simulink model "CounterDroneSystem"  (R2026a)
settings: Solver=FixedStepAuto  StopTime=20  FixedStep=0.001
libraries: simulink x9
settings Model: Creator=ACER  LastModifiedBy=ACER

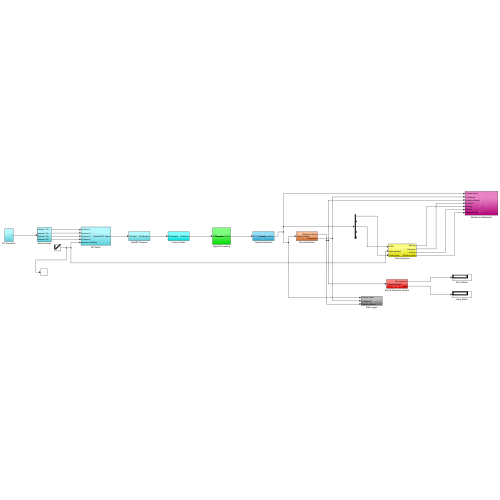
[thumbnail: Simulink's stored preview of the top-level diagram]
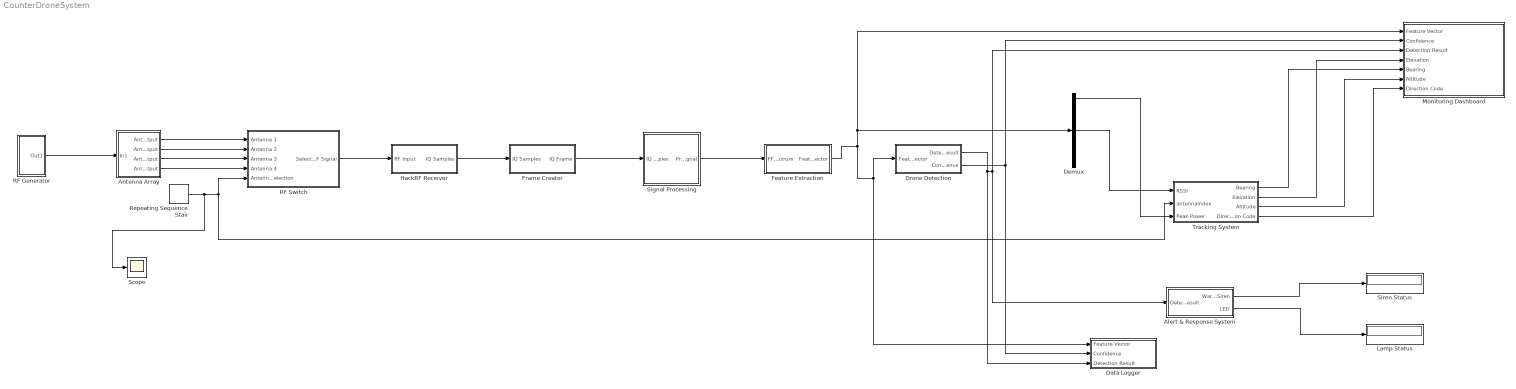
== system CounterDroneSystem ==
  Alert & Response System : Subsystem
  Antenna Array : Subsystem
  Data Logger : Subsystem
  Demux : Demux  Outputs=5
  Drone Detection : Subsystem
  Feature Extraction : Subsystem
  Frame Creator : Subsystem
  HackRF Receiver : Subsystem
  Lamp Status : Display
  Monitoring Dashboard : Subsystem
  RF Generator : Subsystem
  RF Switch : Subsystem
  Repeating Sequence Stair : simulink/Sources/Repeating Sequence Stair  OutValues=[1 2 3 4]  tsamp=5  OutMin=[]  OutMax=[]  OutDataTypeStr=double  OutputDataTypeScalingMode=double  OutDataType=fixdt(0,8)  ConRadixGroup=Best Precision: Vector-wise  OutScaling=2^-12
  Scope : Scope
      settings: ActiveDisplayYMinimum=0.75000000000000011  ActiveDisplayYMaximum=3.25
  Signal Processing : Subsystem
  Siren Status : Display
  Tracking System : Subsystem
  wires:
  RF Generator/1(Out1) -> Antenna Array/1(In1)
  Antenna Array/1(Antenna 1 Output) -> RF Switch/1(Antenna 1)
  Antenna Array/2(Antenna 2 Output) -> RF Switch/2(Antenna 2)
  Signal Processing/1(Processed Signal) -> Feature Extraction/1(FFT Spectrum)
  Feature Extraction/1(Feature Vector) -> Monitoring Dashboard/1(Feature Vector), Demux/1, Data Logger/1(Feature Vector), Drone Detection/1(Feature Vector)
  Drone Detection/2(Confidence) -> Data Logger/2(Confidence), Monitoring Dashboard/2(Confidence)
  Drone Detection/1(Detection Result) -> Data Logger/3(Detection Result), Monitoring Dashboard/3(Detection Result), Alert & Response System/1(Detection Result)
  Tracking System/2(Elevation) -> Monitoring Dashboard/4(Elevation)
  Tracking System/3(" Altitude") -> Monitoring Dashboard/6(Altitude)
  Alert & Response System/1(Warning Siren) -> Siren Status/1
  Alert & Response System/2(" LED") -> Lamp Status/1
  Demux/1 -> Tracking System/3(Peak Power)
  Demux/3 -> Tracking System/1(RSSI)
  Repeating Sequence Stair/1 -> Scope/1, Tracking System/2(antennaIndex), RF Switch/5(Antenna Selection)
  Antenna Array/3(Antenna 3 Output) -> RF Switch/3(Antenna 3)
  Antenna Array/4(Antenna 4 Output) -> RF Switch/4(Antenna 4)
  Frame Creator/1(IQ Frame) -> Signal Processing/1(IQ Samples)
  Tracking System/1(Bearing) -> Monitoring Dashboard/5(Bearing)
  Tracking System/4(Direction Code) -> Monitoring Dashboard/7(Direction Code)
  RF Switch/1(Selected RF Signal) -> HackRF Receiver/1(RF Input)
  HackRF Receiver/1(IQ Samples) -> Frame Creator/1(IQ Samples)

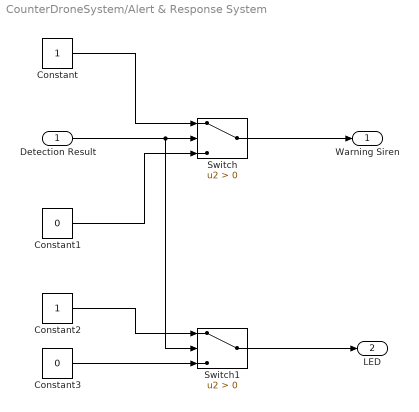
== system CounterDroneSystem/Alert & Response System ==
  Detection Result : Inport
  Constant : Constant
  Constant1 : Constant  Value=0
  Constant2 : Constant
  Constant3 : Constant  Value=0
  Switch : Switch  Criteria=u2 > Threshold  SaturateOnIntegerOverflow=off  InputSameDT=off
  Switch1 : Switch  Criteria=u2 > Threshold  SaturateOnIntegerOverflow=off  InputSameDT=off
  Warning Siren : Outport
  " LED" : Outport  Port=2
  wires:
  Detection Result/1 -> Switch1/2, Switch/2
  Constant/1 -> Switch/1
  Constant1/1 -> Switch/3
  Switch/1 -> Warning Siren/1
  Constant2/1 -> Switch1/1
  Constant3/1 -> Switch1/3
  Switch1/1 -> " LED"/1

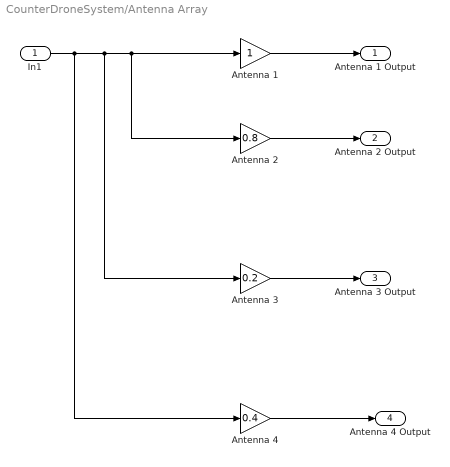
== system CounterDroneSystem/Antenna Array ==
  In1 : Inport
  Antenna 1 : Gain
  Antenna 2 : Gain  Gain=0.8
  Antenna 3 : Gain  Gain=0.2
  Antenna 4 : Gain  Gain=0.4
  Antenna 1 Output : Outport
  Antenna 2 Output : Outport  Port=2
  Antenna 3 Output : Outport  Port=3
  Antenna 4 Output : Outport  Port=4
  wires:
  Antenna 2/1 -> Antenna 2 Output/1
  In1/1 -> Antenna 4/1, Antenna 3/1, Antenna 2/1, Antenna 1/1
  Antenna 1/1 -> Antenna 1 Output/1
  Antenna 3/1 -> Antenna 3 Output/1
  Antenna 4/1 -> Antenna 4 Output/1

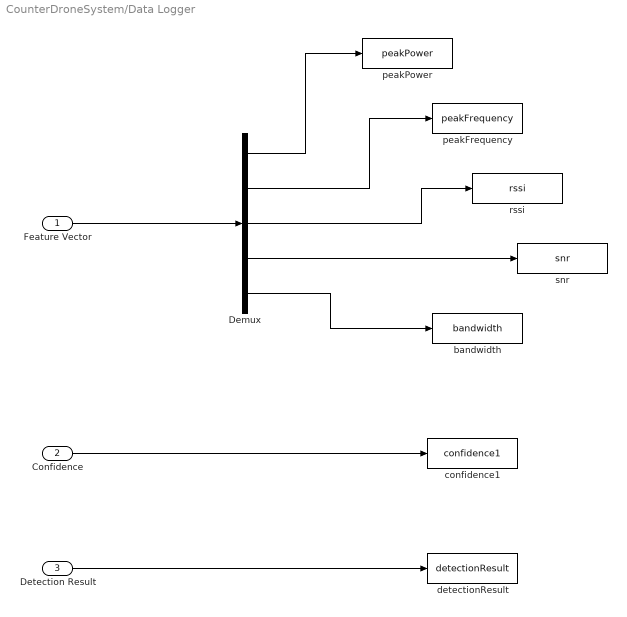
== system CounterDroneSystem/Data Logger ==
  Feature Vector : Inport
  Confidence : Inport  Port=2
  Detection Result : Inport  Port=3
  Demux : Demux  Outputs=5
  bandwidth : ToWorkspace  VariableName=bandwidth  SampleTime=-1
  confidence1 : ToWorkspace  VariableName=confidence1  SampleTime=-1
  detectionResult : ToWorkspace  VariableName=detectionResult  SampleTime=-1
  peakFrequency : ToWorkspace  VariableName=peakFrequency  SampleTime=-1
  peakPower : ToWorkspace  VariableName=peakPower  SampleTime=-1
  rssi : ToWorkspace  VariableName=rssi  SampleTime=-1
  snr : ToWorkspace  VariableName=snr  SampleTime=-1
  wires:
  Feature Vector/1 -> Demux/1
  Demux/1 -> peakPower/1
  Demux/2 -> peakFrequency/1
  Demux/3 -> rssi/1
  Demux/4 -> snr/1
  Demux/5 -> bandwidth/1
  Confidence/1 -> confidence1/1
  Detection Result/1 -> detectionResult/1

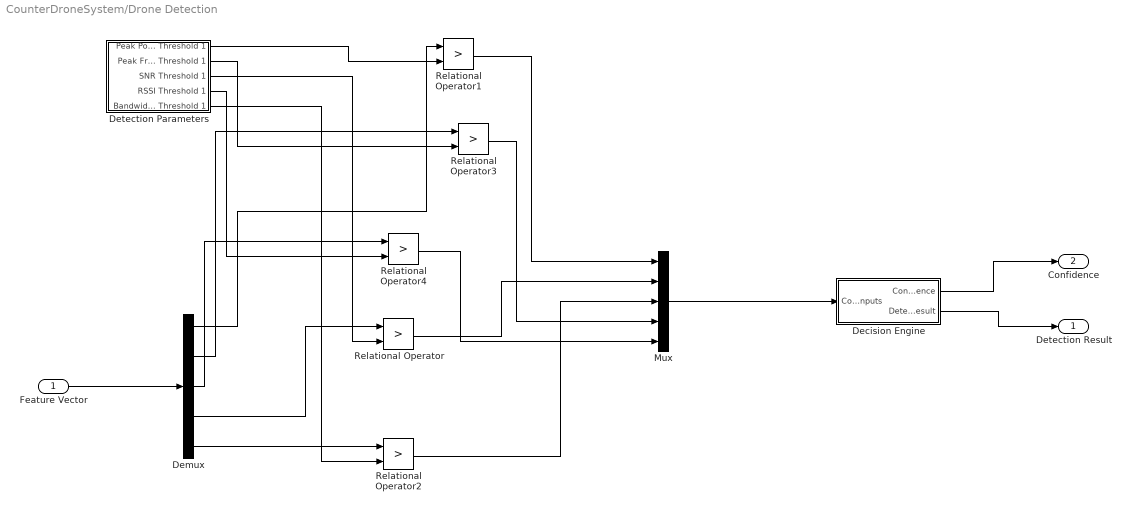
== system CounterDroneSystem/Drone Detection ==
  Feature Vector : Inport
  Decision Engine : Subsystem
  Demux : Demux  Outputs=5
  Detection Parameters : Subsystem
  Mux : Mux  Inputs=5
  Relational Operator{,1..4} (5 alike) : RelationalOperator  Operator=>  OutDataTypeStr=boolean  RndMeth=Simplest  InputSameDT=off
  Detection Result : Outport
  Confidence : Outport  Port=2
  wires:
  Feature Vector/1 -> Demux/1
  Demux/1 -> Relational Operator1/1
  Demux/4 -> Relational Operator/1
  Demux/5 -> Relational Operator2/1
  Relational Operator1/1 -> Mux/1
  Relational Operator/1 -> Mux/2
  Relational Operator2/1 -> Mux/3
  Mux/1 -> Decision Engine/1(Comparator Inputs)
  Decision Engine/1(Confidence) -> Confidence/1
  Decision Engine/2(Detection Result) -> Detection Result/1
  Detection Parameters/1(Peak Power Threshold 1) -> Relational Operator1/2
  Detection Parameters/5(" Bandwidth Threshold 1") -> Relational Operator2/2
  Detection Parameters/3(SNR Threshold 1) -> Relational Operator/2
  Demux/2 -> Relational Operator3/1
  Detection Parameters/2(Peak Frequency Threshold 1) -> Relational Operator3/2
  Relational Operator3/1 -> Mux/4
  Relational Operator4/1 -> Mux/5
  Detection Parameters/4(RSSI Threshold 1) -> Relational Operator4/2
  Demux/3 -> Relational Operator4/1

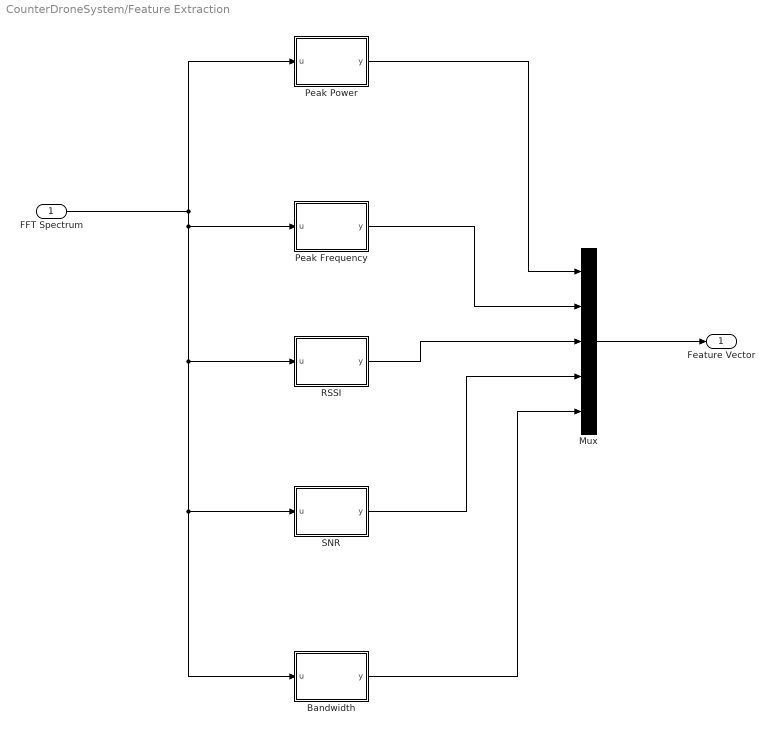
== system CounterDroneSystem/Feature Extraction ==
  FFT Spectrum : Inport
  Bandwidth : MATLAB Function  TreatAsAtomicUnit=on
  Mux : Mux  Inputs=5
  Peak Frequency : MATLAB Function  TreatAsAtomicUnit=on
  Peak Power : MATLAB Function  TreatAsAtomicUnit=on
  RSSI : MATLAB Function  TreatAsAtomicUnit=on
  SNR : MATLAB Function  TreatAsAtomicUnit=on
  Feature Vector : Outport
  wires:
  FFT Spectrum/1 -> Peak Frequency/1(u), Bandwidth/1(u), SNR/1(u), RSSI/1(u), Peak Power/1(u)
  Mux/1 -> Feature Vector/1
  RSSI/1(y) -> Mux/3
  SNR/1(y) -> Mux/4
  Bandwidth/1(y) -> Mux/5
  Peak Frequency/1(y) -> Mux/2
  Peak Power/1(y) -> Mux/1

== system CounterDroneSystem/Frame Creator ==
  IQ Samples : Inport
  Buffer : Buffer  N=256  OutputFrames=off
  IQ Frame : Outport
  wires:
  IQ Samples/1 -> Buffer/1
  Buffer/1 -> IQ Frame/1

== system CounterDroneSystem/HackRF Receiver ==
  RF Input : Inport
  LNA : Gain  Gain=10
  IQ Samples : Outport
  wires:
  RF Input/1 -> LNA/1
  LNA/1 -> IQ Samples/1

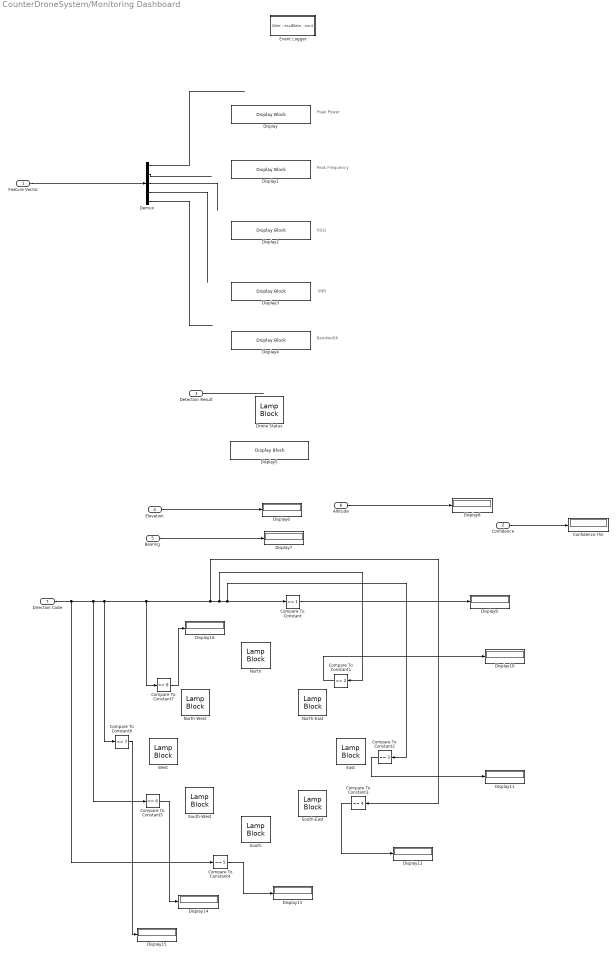
== system CounterDroneSystem/Monitoring Dashboard ==
  note: Peak Frequency
  note: Bandwidth
  note: SNR
  note: Peak Power
  note: RSSI
  Feature Vector : Inport
  Confidence : Inport  Port=2
  Detection Result : Inport  Port=3
  Elevation : Inport  Port=4
  Bearing : Inport  Port=5
  Altitude : Inport  Port=6
  Direction Code : Inport  Port=7
  " Confidence (%)" : Display
  Compare To Constant : simulink/Logic and Bit Operations/Compare To Constant  relop===  const=1  OutDataTypeStr=boolean
  Compare To Constant1 : simulink/Logic and Bit Operations/Compare To Constant  relop===  const=2  OutDataTypeStr=boolean
  Compare To Constant2 : simulink/Logic and Bit Operations/Compare To Constant  relop===  const=3  OutDataTypeStr=boolean
  Compare To Constant3 : simulink/Logic and Bit Operations/Compare To Constant  relop===  const=4  OutDataTypeStr=boolean
  Compare To Constant4 : simulink/Logic and Bit Operations/Compare To Constant  relop===  const=5  OutDataTypeStr=boolean
  Compare To Constant5 : simulink/Logic and Bit Operations/Compare To Constant  relop===  const=6  OutDataTypeStr=boolean
  Compare To Constant6 : simulink/Logic and Bit Operations/Compare To Constant  relop===  const=7  OutDataTypeStr=boolean
  Compare To Constant7 : simulink/Logic and Bit Operations/Compare To Constant  relop===  const=8  OutDataTypeStr=boolean
  Demux : Demux  Outputs=5
  Display{,1..5} (6 alike) : DisplayBlock  LabelPosition=Hide  Transparency=1  GridColor=[0.502, 0.502, 0.502]
  Display{6..16} (11 alike) : Display
  Drone Status : LampBlock  LabelPosition=Hide  DefaultColor=[192.0, 192.0, 192.0]
  East : LampBlock  LabelPosition=Hide  DefaultColor=[192.0, 192.0, 192.0]
  Event Logger : Subsystem
  North : LampBlock  LabelPosition=Hide  DefaultColor=[192.0, 192.0, 192.0]
  North-East : LampBlock  LabelPosition=Hide  DefaultColor=[192.0, 192.0, 192.0]
  North-West : LampBlock  LabelPosition=Hide  DefaultColor=[192.0, 192.0, 192.0]
  South : LampBlock  LabelPosition=Hide  DefaultColor=[192.0, 192.0, 192.0]
  South-East : LampBlock  LabelPosition=Hide  DefaultColor=[192.0, 192.0, 192.0]
  South-West : LampBlock  LabelPosition=Hide  DefaultColor=[192.0, 192.0, 192.0]
  West : LampBlock  LabelPosition=Hide  DefaultColor=[192.0, 192.0, 192.0]
  wires:
  Demux/2 -> ?
  Demux/1 -> ?
  Demux/5 -> ?
  Demux/3 -> ?
  Demux/4 -> ?
  Feature Vector/1 -> Demux/1
  Confidence/1 -> " Confidence (%)"/1
  Detection Result/1 -> ?
  Elevation/1 -> Display6/1
  Bearing/1 -> Display7/1
  Altitude/1 -> Display8/1
  Direction Code/1 -> Compare To Constant4/1, Compare To Constant5/1, Compare To Constant3/1, Compare To Constant1/1, Compare To Constant2/1, Compare To Constant/1, Compare To Constant7/1, Compare To Constant6/1
  Compare To Constant/1 -> Display9/1
  Compare To Constant1/1 -> Display10/1
  Compare To Constant2/1 -> Display11/1
  Compare To Constant3/1 -> Display12/1
  Compare To Constant4/1 -> Display13/1
  Compare To Constant5/1 -> Display14/1
  Compare To Constant6/1 -> Display15/1
  Compare To Constant7/1 -> Display16/1

== system CounterDroneSystem/RF Generator ==
  Random Number : RandomNumber  Variance=0.01  SampleTime=0.001
  Sine Wave : Sin  Amplitude=10  Frequency=1000  SampleTime=0.001
  Sum : Sum  Inputs=|++
  Out1 : Outport
  wires:
  Sine Wave/1 -> Sum/1
  Sum/1 -> Out1/1
  Random Number/1 -> Sum/2

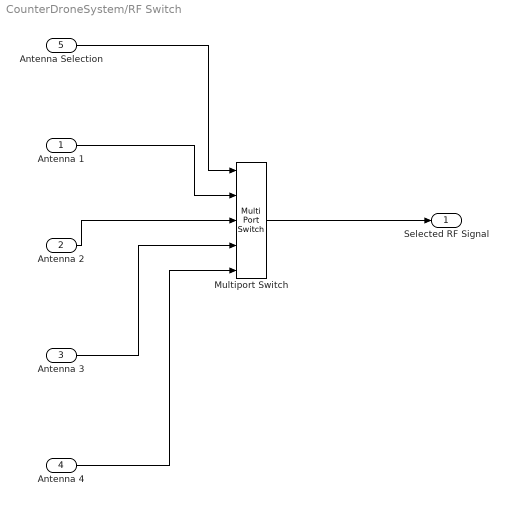
== system CounterDroneSystem/RF Switch ==
  Antenna 1 : Inport
  Antenna 2 : Inport  Port=2
  Antenna 3 : Inport  Port=3
  Antenna 4 : Inport  Port=4
  Antenna Selection : Inport  Port=5
  Multiport Switch : MultiPortSwitch  Inputs=4  SaturateOnIntegerOverflow=off  InputSameDT=off
  Selected RF Signal : Outport
  wires:
  Antenna Selection/1 -> Multiport Switch/1
  Antenna 1/1 -> Multiport Switch/2
  Antenna 2/1 -> Multiport Switch/3
  Antenna 3/1 -> Multiport Switch/4
  Antenna 4/1 -> Multiport Switch/5
  Multiport Switch/1 -> Selected RF Signal/1

== system CounterDroneSystem/Signal Processing ==
  IQ Samples : Inport
  Array Plot : ArrayPlot  WindowPosition=[19.000000,179.000000,800.000000,500.000000,]  ScopeFrameLocation=window  AxesScaling=Manual  Title=RF Power Spectrum  YLimits=[-529.6101893004114 1954.8544106995882]
  Band Pass Filter : Subsystem
  Power Estimation : MATLAB Function  TreatAsAtomicUnit=on
  Processed Signal : Outport
  wires:
  IQ Samples/1 -> Band Pass Filter/1(IQ Samples)
  Band Pass Filter/1(FFT Spectrum) -> Power Estimation/1(u)
  Power Estimation/1(y) -> Array Plot/1, Processed Signal/1

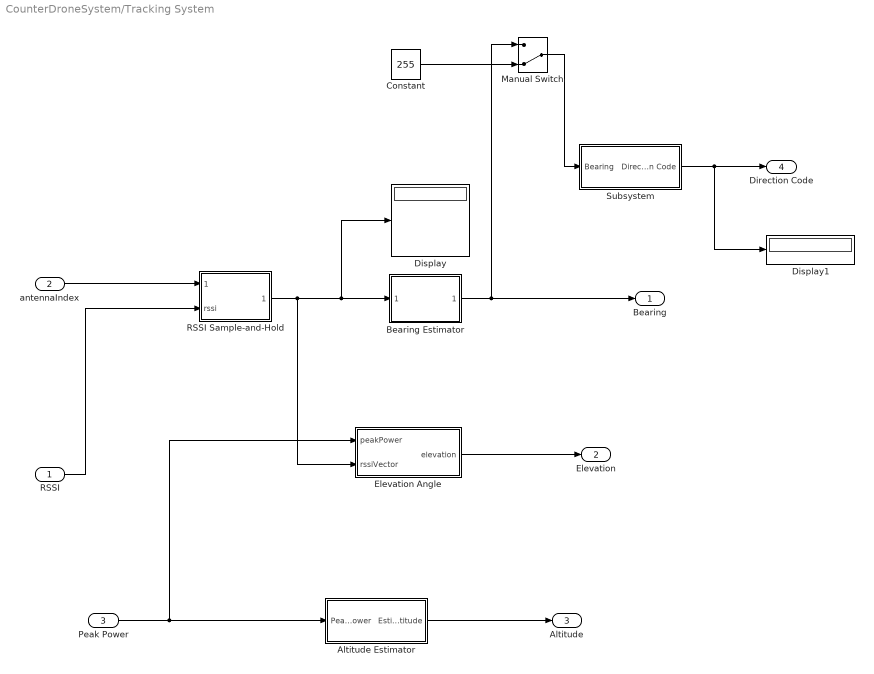
== system CounterDroneSystem/Tracking System ==
  RSSI : Inport
  antennaIndex : Inport  Port=2
  Peak Power : Inport  Port=3
  Altitude Estimator : Subsystem
  Bearing Estimator : MATLAB Function  TreatAsAtomicUnit=on
  Constant : Constant  Value=255
  Display : Display
  Display1 : Display
  Elevation Angle : MATLAB Function  TreatAsAtomicUnit=on
  Manual Switch : ManualSwitch  CurrentSetting=0
  RSSI Sample-and-Hold : MATLAB Function  TreatAsAtomicUnit=on
  Subsystem : Subsystem
  Bearing : Outport
  Elevation : Outport  Port=2
  " Altitude" : Outport  Port=3
  Direction Code : Outport  Port=4
  wires:
  Altitude Estimator/1(Estimated Altitude) -> " Altitude"/1
  Peak Power/1 -> Elevation Angle/1(peakPower), Altitude Estimator/1(Peak power)
  antennaIndex/1 -> RSSI Sample-and-Hold/1(antennaIndex)
  RSSI/1 -> RSSI Sample-and-Hold/2(rssi)
  RSSI Sample-and-Hold/1(rssiVector) -> Elevation Angle/2(rssiVector), Display/1, Bearing Estimator/1(rssiVector)
  Bearing Estimator/1(bearing) -> Bearing/1, Manual Switch/1
  Elevation Angle/1(elevation) -> Elevation/1
  Subsystem/1(Direction Code) -> Display1/1, Direction Code/1
  Constant/1 -> Manual Switch/2
  Manual Switch/1 -> Subsystem/1(Bearing)

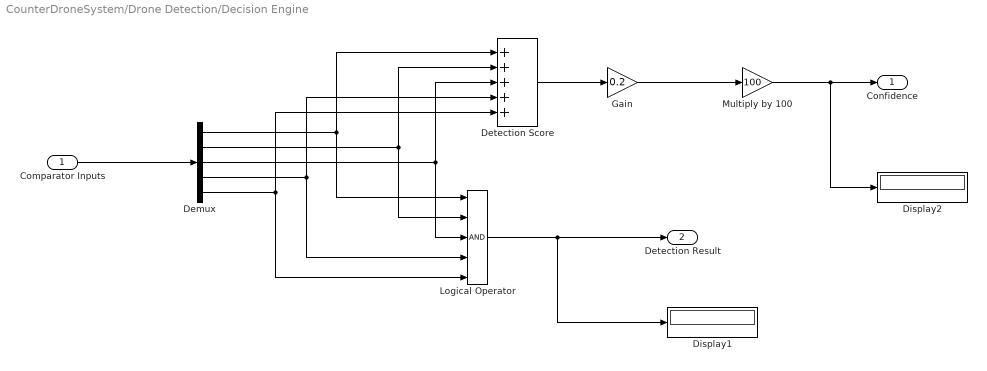
== system CounterDroneSystem/Drone Detection/Decision Engine ==
  Comparator Inputs : Inport
  Demux : Demux  Outputs=5
  Detection Score : Sum  Inputs=+++++
  Display1 : Display
  Display2 : Display
  Gain : Gain  Gain=0.2
  Logical Operator : Logic  Inputs=5  AllPortsSameDT=off  OutDataTypeStr=boolean
  Multiply by 100 : Gain  Gain=100
  Confidence : Outport
  Detection Result : Outport  Port=2
  wires:
  Multiply by 100/1 -> Display2/1, Confidence/1
  Demux/3 -> Logical Operator/3, Detection Score/3
  Logical Operator/1 -> Display1/1, Detection Result/1
  Gain/1 -> Multiply by 100/1
  Demux/2 -> Logical Operator/2, Detection Score/2
  Detection Score/1 -> Gain/1
  Demux/1 -> Logical Operator/1, Detection Score/1
  Comparator Inputs/1 -> Demux/1
  Demux/4 -> Logical Operator/4, Detection Score/4
  Demux/5 -> Logical Operator/5, Detection Score/5

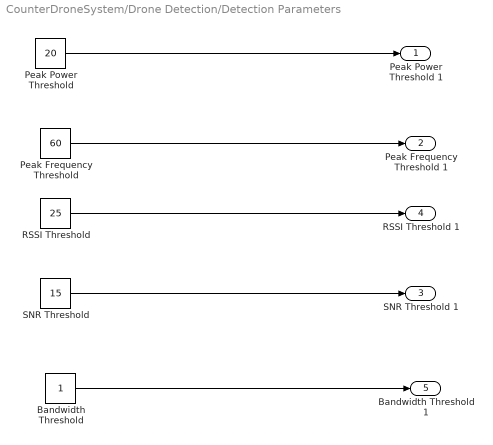
== system CounterDroneSystem/Drone Detection/Detection Parameters ==
  Bandwidth Threshold : Constant
  Peak Frequency Threshold : Constant  Value=60
  Peak Power Threshold : Constant  Value=20
  RSSI Threshold : Constant  Value=25
  SNR Threshold : Constant  Value=15
  Peak Power Threshold 1 : Outport
  Peak Frequency Threshold 1 : Outport  Port=2
  SNR Threshold 1 : Outport  Port=3
  RSSI Threshold 1 : Outport  Port=4
  " Bandwidth Threshold 1" : Outport  Port=5
  wires:
  Peak Power Threshold/1 -> Peak Power Threshold 1/1
  RSSI Threshold/1 -> RSSI Threshold 1/1
  SNR Threshold/1 -> SNR Threshold 1/1
  Bandwidth Threshold/1 -> " Bandwidth Threshold 1"/1
  Peak Frequency Threshold/1 -> Peak Frequency Threshold 1/1

== system CounterDroneSystem/Monitoring Dashboard/Event Logger ==
  Detection Result : Inport
  Detection Count : Outport
  wires:
  Detection Result/1 -> Detection Count/1

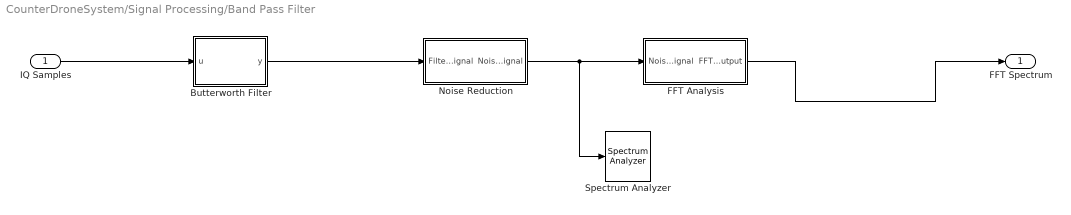
== system CounterDroneSystem/Signal Processing/Band Pass Filter ==
  IQ Samples : Inport
  Butterworth Filter : MATLAB Function  TreatAsAtomicUnit=on
  FFT Analysis : Subsystem
  Noise Reduction : Subsystem
  Spectrum Analyzer : SpectrumAnalyzer  WindowPosition=[1.000000,1.000000,1536.000000,841.000000,]  Visible=on  ScopeFrameLocation=window  WindowInvariantSamplesPerUpdate=on  Span=1000  StartFrequency=-500  StopFrequency=500  YLimits=[-35.2084 48.8632]
  FFT Spectrum : Outport
  wires:
  IQ Samples/1 -> Butterworth Filter/1(u)
  Butterworth Filter/1(y) -> Noise Reduction/1(Filtered Signal)
  Noise Reduction/1(Noise Reduced Signal) -> Spectrum Analyzer/1, FFT Analysis/1(Noise Reduced Signal)
  FFT Analysis/1(FFT Output) -> FFT Spectrum/1

== system CounterDroneSystem/Tracking System/Altitude Estimator ==
  Peak power : Inport
  Bias : Bias  Bias=0.05  SaturateOnIntegerOverflow=off
  Gain : Gain  Gain=0.5
  Saturation : Saturate  UpperLimit=120  LowerLimit=0
  Estimated Altitude : Outport
  wires:
  Peak power/1 -> Gain/1
  Gain/1 -> Bias/1
  Bias/1 -> Saturation/1
  Saturation/1 -> Estimated Altitude/1

== system CounterDroneSystem/Tracking System/Subsystem ==
  Bearing : Inport
  MATLAB Function : MATLAB Function  TreatAsAtomicUnit=on
  Direction Code : Outport
  wires:
  Bearing/1 -> MATLAB Function/1(bearing)
  MATLAB Function/1(direction) -> Direction Code/1

== system CounterDroneSystem/Signal Processing/Band Pass Filter/FFT Analysis ==
  Noise Reduced Signal : Inport
  FFT Processor : MATLAB Function  TreatAsAtomicUnit=on
  FFT Output : Outport
  wires:
  Noise Reduced Signal/1 -> FFT Processor/1(u)
  FFT Processor/1(y) -> FFT Output/1

== system CounterDroneSystem/Signal Processing/Band Pass Filter/Noise Reduction ==
  Filtered Signal : Inport
  Noise Reduction : MATLAB Function  TreatAsAtomicUnit=on
  Noise Reduced Signal : Outport
  wires:
  Filtered Signal/1 -> Noise Reduction/1(u)
  Noise Reduction/1(y) -> Noise Reduced Signal/1

== matlab function CounterDroneSystem/Signal Processing/Band Pass Filter/Butterworth Filter ==
  data: u input; y output
function y = fcn(u)
%--------------------------------------------------------------------------
% Counter Drone System
% Band Pass Filter
%
% Input  : u  -> IQ Samples
% Output : y  -> Filtered Signal
%
% Current Version:
% Passes the signal directly.
% A real Butterworth Band Pass Filter will be added later.
%--------------------------------------------------------------------------

% Pass the input signal directly
y = u;

end

== matlab function CounterDroneSystem/Signal Processing/Band Pass Filter/FFT Analysis/FFT Processor ==
  data: u input; y output
function y = fcn(u)
%=========================================================
% Counter Drone System
% FFT Processor
%
% Input  : IQ Samples
% Output : Normalized FFT Magnitude Spectrum
%=========================================================

% Convert to column vector
x = u(:);

% Number of samples
N = length(x);

% Compute normalized FFT
X = fft(x)/N;

% Shift zero frequency to center
X = fftshift(X);

% Magnitude spectrum
y = abs(X);

end

== matlab function CounterDroneSystem/Signal Processing/Power Estimation ==
  data: u input; y output
function y = fcn(u)

% Power Spectrum

y = abs(u).^2;

% Remove DC component
y = y - min(y);

end

== matlab function CounterDroneSystem/Tracking System/Subsystem/MATLAB Function ==
  data: bearing input; direction output
function direction = fcn(bearing)

bearing = mod(bearing,360);

if bearing >= 337.5 || bearing < 22.5
    direction = 1;      % North

elseif bearing >=22.5 && bearing <67.5
    direction = 2;      % North-East

elseif bearing >=67.5 && bearing <112.5
    direction = 3;      % East

elseif bearing >=112.5 && bearing <157.5
    direction = 4;      % South-East

elseif bearing >=157.5 && bearing <202.5
    direction = 5;      % South

elseif bearing >=202.5 && bearing <247.5
    direction = 6;      % South-West

elseif bearing >=247.5 && bearing <292.5
    direction = 7;      % West

else
    direction = 8;      % North-West

end

== matlab function CounterDroneSystem/Feature Extraction/Peak Power ==
  data: u input; y output
function y = fcn(u)

% Peak Power in dB

peak = max(u);

y = 10*log10(peak + eps);

end

== matlab function CounterDroneSystem/Feature Extraction/Peak Frequency ==
  data: u input; y output
function y = fcn(u)

[~,idx] = max(abs(u));
y = idx;

end

== matlab function CounterDroneSystem/Feature Extraction/RSSI ==
  data: u input; y output
function y = fcn(u)

y = 10*log10(mean(abs(u).^2)+eps);

end

== matlab function CounterDroneSystem/Feature Extraction/SNR ==
  data: u input; y output
function y = fcn(u)

signal = max(abs(u).^2);
noise = mean(abs(u).^2);

y = 10*log10(signal/(noise+eps));

end

== matlab function CounterDroneSystem/Feature Extraction/Bandwidth ==
  data: u input; y output
function y = fcn(u)

threshold = max(abs(u))*0.5;

index = find(abs(u)>threshold);

y = length(index);

end

== matlab function CounterDroneSystem/Tracking System/RSSI Sample-and-Hold ==
  data: antennaIndex input; rssiVector output; rssi input
function rssiVector = fcn(antennaIndex, rssi)
persistent heldValues lastIndex skipCount
if isempty(heldValues)
    heldValues = zeros(1,4);
    lastIndex = -1;
    skipCount = 0;
end
idx = round(antennaIndex);
if idx ~= lastIndex
    lastIndex = idx;
    skipCount = 2;
end
if idx >= 1 && idx <= 4
    if skipCount > 0
        skipCount = skipCount - 1;
    else
        heldValues(idx) = rssi;
    end
end
rssiVector = heldValues;
end

== matlab function CounterDroneSystem/Signal Processing/Band Pass Filter/Noise Reduction/Noise Reduction ==
  data: u input; y output
function y = fcn(u)
%---------------------------------------------------------
% Counter Drone System
% Noise Reduction
%
% Input  : Filtered Signal
% Output : Noise Reduced Signal
%
% Current Version:
% Passes the signal directly.
% A real denoising algorithm will be added later.
%---------------------------------------------------------

% Pass input directly to output
y = u;

end

== matlab function CounterDroneSystem/Tracking System/Bearing Estimator ==
  data: rssiVector input; bearing output
function bearing = fcn(rssiVector)
angles = [0 90 180 270];
linPower = 10.^(rssiVector/10);
[~, maxIdx] = max(linPower);
leftIdx  = mod(maxIdx-2,4) + 1;
rightIdx = mod(maxIdx,4) + 1;
if linPower(leftIdx) >= linPower(rightIdx)
    neighborIdx = leftIdx;
else
    neighborIdx = rightIdx;
end
w1 = linPower(maxIdx);
w2 = linPower(neighborIdx);
a1 = angles(maxIdx);
a2 = angles(neighborIdx);
diffAngle = a2 - a1;
if diffAngle > 180
    diffAngle = diffAngle - 360;
elseif diffAngle < -180
    diffAngle = diffAngle + 360;
end
fraction = w2 / (w1 + w2 + eps);
bearing = mod(a1 + fraction*diffAngle, 360);
end

== matlab function CounterDroneSystem/Tracking System/Elevation Angle ==
  data: peakPower input; elevation output double; rssiVector input
function elevation = fcn(peakPower, rssiVector)

validRSSI = rssiVector(rssiVector ~= 0);

if numel(validRSSI) < 2
    elevation = 0;
    return;
end

rssiStd = std(double(validRSSI));

maxStd = 15;

elevation = 90*(1 - rssiStd/maxStd);

elevation = max(0,min(90,elevation));

end
